simulink model "cartBrick_simulink"  (R2025b)
settings: Solver=ode45  StartTime=0.0  StopTime=10  RelTol=1e-3
values from neighbouring files (symbols this model uses):
  N = 20    [cart_brick_ocp.m]
  nu = length(model.u)    [cart_brick_ocp.m]
undefined symbols (not defined in the file or in its folder): X, Y, Z
libraries: sm_lib x14, nesl_utility x7, simulink x1
settings Model: Creator=oj  LastModifiedBy=itsan
settings SolverCC: AlgebraicLoopSolver=TrustRegion
settings DataIOCC: SaveFormat=StructureWithTime
settings OptimizationCC: LifeSpan=inf
settings DebuggingCC: UnconnectedInputMsg=warning  UnconnectedOutputMsg=warning  UnconnectedLineMsg=warning  SFExecutionAtInitializationDiag=none  ArithmeticOperatorsInVariantConditions=warning
settings HardwareCC: ProdBitPerSizeT=32.0  ProdBitPerPtrDiffT=32.0  ProdWordSize=32.0  ProdHWDeviceType=Specified
settings SFSimCC: CustomCodeUndefinedFunction=UseInterfaceOnly
settings RTWCC: GPUComputeCapability=3.5
settings CodeAppCC: StateflowObjectComments=on

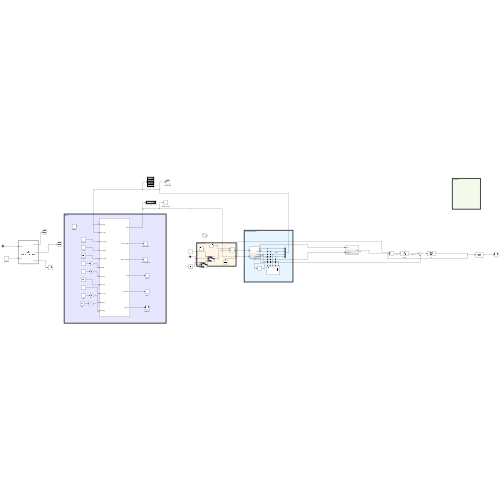
[thumbnail: Simulink's stored preview of the top-level diagram]
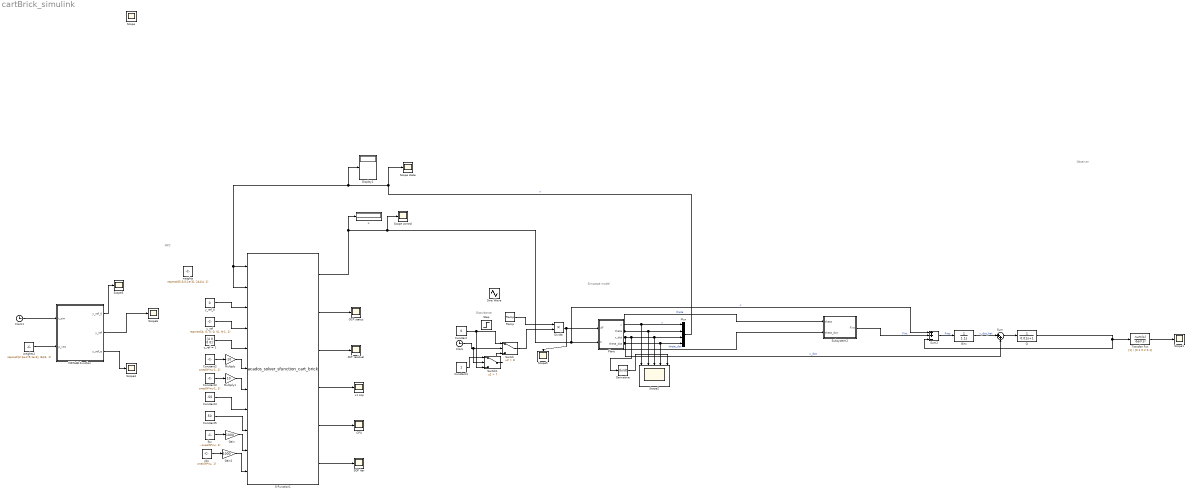
== system cartBrick_simulink ==
  note: Simscape model
  note: Observer
  note: Disturbance
  note: MPC
  CPU : Scope
      settings: Description=status  ActiveDisplayYMinimum=4.7875000000000012E-5  ActiveDisplayYMaximum=0.000858125  DataLoggingVariableName=ScopeData3
  Clock : Clock
      settings: Decimation=7
  Clock1 : Clock
  Constant : Constant  Value=0
  Constant1 : Constant
  Constant2 : Constant  Value=ones(N*nu-1, 1)
  Constant3 : Constant  Value=ones(N*nu-1, 1)
  Constant4 : Constant  Value=-50
  Constant5 : Constant  Value=50
  Derivative : Derivative
  Display1 : Display
  Divide : Product  Inputs=**
  Gain : Gain  Gain=1000
  Gain1 : Gain  Gain=1000
  Ginv : TransferFcn  Denominator=[1.1 0]
  KKT residual : Scope
      settings: Description=status  ActiveDisplayYMinimum=-0.32883901659053916  ActiveDisplayYMaximum=1.592767698176573  DataLoggingVariableName=ScopeData4
  MATLAB Function : MATLAB Function  TreatAsAtomicUnit=on
  Multiply : Gain  Gain=-10
  Multiply1 : Gain  Gain=10
  Mux : Mux
  OCP status : Scope
      settings: Description=status  ActiveDisplayYMinimum=-2.0851401210050069  ActiveDisplayYMaximum=5.2280116787993132
  Plant : Subsystem
  Q : TransferFcn  Denominator=[0.01 1]
  Ramp : simulink/Sources/Ramp  slope=1  start=1  InitialOutput=0
  S-Function1 : S-Function  FunctionName=acados_solver_sfunction_cart_brick  SFunctionDeploymentMode=off  EnableBusSupport=off
      mask Display:
      | % from the make_sfun file
      | global sfun_input_names sfun_output_names
      | for i = 1:length(sfun_input_names)
      | 	port_label('input', i, sfun_input_names{i})
      | end
      | for i = 1:length(sfun_output_names)
      | 	port_label('output', i, sfun_output_names{i})
      | end
  SQP iter : Scope
      settings: Description=status  ActiveDisplayYMinimum=0.875  ActiveDisplayYMaximum=2.125  DataLoggingVariableName=ScopeData5
  Scope control : Scope
      settings: ActiveDisplayYMinimum=-505.22988338563073  ActiveDisplayYMaximum=1195.552745234269  DataLoggingVariableName=ScopeData6
  Scope state : Scope
      settings: ActiveDisplayYMinimum=-0.21964245596561607  ActiveDisplayYMaximum=0.1960092178367589  DataLoggingVariableName=ScopeData7
  Scope{,1,3..6} (6 alike) : Scope
      Scope1 settings: ActiveDisplayYMinimum=-1  ActiveDisplayYMaximum=1  DataLoggingVariableName=ScopeData8
      Scope3 settings: ActiveDisplayYMinimum=-1.7541433017886874  ActiveDisplayYMaximum=4.946334901336316  DataLoggingVariableName=ScopeData10
      Scope4 settings: ActiveDisplayYMinimum=-1.7541433017886874  ActiveDisplayYMaximum=4.946334901336316  DataLoggingVariableName=ScopeData11
      Scope5 settings: ActiveDisplayYMinimum=-1.183238458570643  ActiveDisplayYMaximum=1.630962386741857  DataLoggingVariableName=ScopeData12
      Scope6 settings: ActiveDisplayYMinimum=-1.7541433017886874  ActiveDisplayYMaximum=4.946334901336316  DataLoggingVariableName=ScopeData13
      Scope settings: ActiveDisplayYMinimum=-13.79726  ActiveDisplayYMaximum=10.28583
  Scope2 : Scope  NumInputPorts=5
      settings: ActiveDisplayYMinimum=-14.024186405885914  ActiveDisplayYMaximum=38.526811919180453  DataLoggingVariableName=ScopeData9
  Sine Wave : Sin  Frequency=6*pi  SampleTime=0
  Step : Step  Before=3  After=0  SampleTime=0
  Subsystem2 : Subsystem
  Sum : Sum  Inputs=|++
  Sum2 : Sum  Inputs=+|+|-
  Switch : Switch  Criteria=u2 > Threshold  Threshold=8  SaturateOnIntegerOverflow=off  InputSameDT=off
  Switch1 : Switch  Criteria=u2 > Threshold  Threshold=7  SaturateOnIntegerOverflow=off  InputSameDT=off
  Transfer Fcn : TransferFcn  Denominator=[0.1 0.2 0.1]
  lbu : Constant  Value=- ones(N*nu, 1)
  u : Display
  ubu : Constant  Value=ones(N*nu, 1)
  weights : Constant  Value=repmat([5;3;0;1e-3], 244/4, 1)
  weights1 : Constant  Value=repmat([2;1e-2;5;1e-2], 84/4, 1)
  x1 ocp : Scope
      settings: Description=status  ActiveDisplayYMinimum=-2.6422889921421415  ActiveDisplayYMaximum=2.2266101006407979  DataLoggingVariableName=ScopeData2
  y_ref : Constant  Value=repmat([4; 0; 0; 0; 0], N-1, 1)
  y_ref = 1 : Constant  Value=[4 0 0 0]'
  y_ref_0 : Constant  Value=0
  wires:
  S-Function1/5 -> CPU/1
  S-Function1/6 -> SQP iter/1
  S-Function1/3 -> KKT residual/1
  Mux/1 -> Display1/1, S-Function1/2, S-Function1/1, Scope state/1  "x"
  lbu/1 -> Gain/1
  S-Function1/4 -> x1 ocp/1
  S-Function1/2 -> OCP status/1
  Plant/1(x) -> Mux/1, Scope2/1  "x"
  Plant/3(x_dot) -> Sum/2, Derivative/1, Mux/3, Scope2/3  "x_dot"
  Clock/1 -> Switch1/2, Switch/2
  Constant/1 -> Switch1/3, Switch/1
  Divide/1 -> Plant/1(dF), Scope5/1
  Switch/1 -> Divide/2
  ubu/1 -> Gain1/1
  Constant2/1 -> Multiply/1
  Constant3/1 -> Multiply1/1
  Plant/2(theta) -> Subsystem2/1(theta), Mux/2, Scope2/2  "theta"
  S-Function1/1 -> u/1, Sum2/1, Plant/2(F), Scope control/1  "u"
  Plant/4(theta_dot) -> Subsystem2/2(theta_dot), Mux/4, Scope2/4  "theta_dot"
  Subsystem2/1(Fint) -> Sum2/2  "Fint"
  Q/1 -> Transfer Fcn/1, Sum2/3
  Sum2/1 -> Ginv/1  "Fres"
  Ginv/1 -> Sum/1  "x_dot_hat"
  Sum/1 -> Q/1
  Transfer Fcn/1 -> Scope1/1
  Derivative/1 -> Scope2/5
  Switch1/1 -> Switch/3
  Constant1/1 -> Switch1/1
  Clock1/1 -> MATLAB Function/1(t_sim)
  MATLAB Function/1(y_ref_0) -> Scope3/1
  MATLAB Function/2(y_ref) -> Scope6/1
  MATLAB Function/3(y_ref_e) -> Scope4/1
  weights1/1 -> MATLAB Function/2(p_vec)
  Gain1/1 -> S-Function1/11
  Gain/1 -> S-Function1/10
  Constant5/1 -> S-Function1/9
  Constant4/1 -> S-Function1/8
  Multiply1/1 -> S-Function1/7
  Multiply/1 -> S-Function1/6
  y_ref = 1/1 -> S-Function1/5
  y_ref_0/1 -> S-Function1/3
  y_ref/1 -> S-Function1/4
  Ramp/1 -> Divide/1

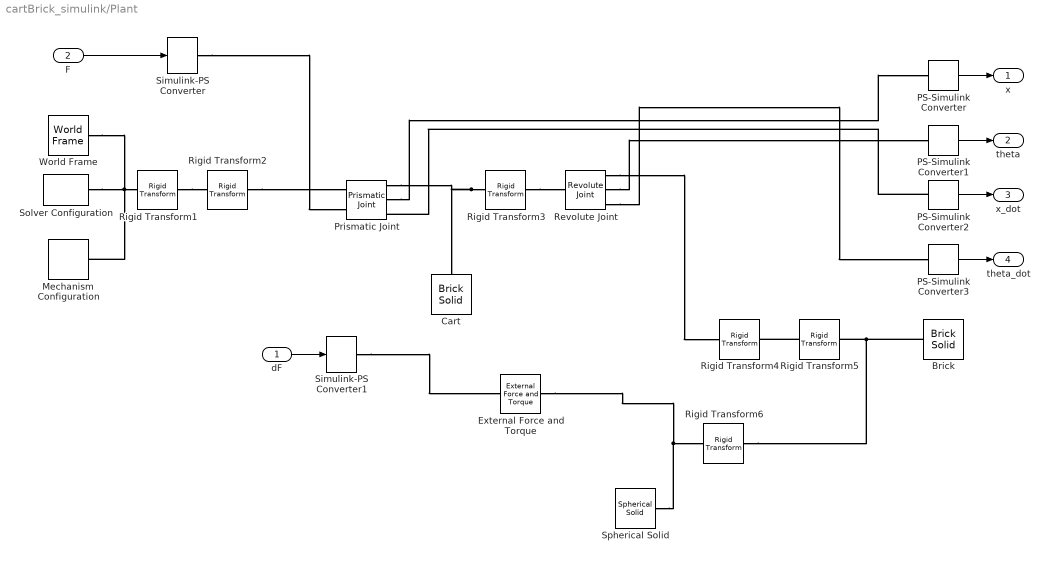
== system cartBrick_simulink/Plant ==
  dF : Inport
  F : Inport  Port=2
  Brick : sm_lib/Body Elements/Brick Solid  BrickDimensions=[0.3 0.8 1]  BrickDimensionsUnits=m  ExportEntireGeometry=off  InertiaType=CalculateFromGeometry  BasedOnType=Mass  Density=1000  DensityUnits=kg/(m^3)  Mass=6  MassUnits=kg  CenterOfMass=[0 0 0]  CenterOfMassUnits=m  MomentsOfInertia=[1 1 1]  MomentsOfInertiaUnits=kg*m^2  ProductsOfInertia=[0 0 0]  ProductsOfInertiaUnits=kg*m^2  GraphicType=FromGeometry  MarkerShape=Sphere  MarkerSize=10  GraphicVisPropType=SimpleVisualProperties  GraphicDiffuseColor=[0.8 0.0 0.2]  GraphicOpacity=0.6  GraphicSpecularColor=[0.5 0.5 0.5 1.0]  GraphicAmbientColor=[0.15 0.15 0.15 1.0]  GraphicEmissiveColor=[0.0 0.0 0.0 1.0]  GraphicShininess=75  DoExposeReferenceFrame=off  SerializedFrames=|
      | <Frames>
      | 
      |   <Frame>
      |     <Id>Frame2</Id>
      |     <Value>
      |       <Name>B</Name>
      |       <Origin>
      |         <Source>GeometricFeature</Source>
      |         <FeatureName>-z surface</FeatureName>
      |       </Origin>
      |       <PrimaryAxis>
      |         <DefinedDirection>+Z</DefinedDirection>
      |         <Source>ReferenceFrame</Source>
      |         <SourceDirection>+Z</SourceDirection>
      |         <FeatureName></FeatureName>
      |       </PrimaryAxis>
      |       <SecondaryAxis>
      |         <DefinedDirection>+X</DefinedDirection>
      |         <Source>ReferenceFrame</Source>
      |         <SourceDirection>+X</SourceDirection>
      |         <FeatureName></FeatureName>
      |       </SecondaryAxis>
      |     </Value>
      |   </Frame>
      | 
      | </Frames>
  Cart : sm_lib/Body Elements/Brick Solid  BrickDimensions=[0.3 0.3 0.3]  BrickDimensionsUnits=m  ExportEntireGeometry=off  InertiaType=PointMass  BasedOnType=Mass  Density=1000  DensityUnits=kg/(m^3)  Mass=10  MassUnits=kg  CenterOfMass=[0 0 0]  CenterOfMassUnits=m  MomentsOfInertia=[1 1 1]  MomentsOfInertiaUnits=kg*m^2  ProductsOfInertia=[0 0 0]  ProductsOfInertiaUnits=kg*m^2  GraphicType=FromGeometry  MarkerShape=Sphere  MarkerSize=10  GraphicVisPropType=SimpleVisualProperties  GraphicDiffuseColor=[0.5 0.5 0.5]  GraphicOpacity=0.5  GraphicSpecularColor=[0.5 0.5 0.5 1.0]  GraphicAmbientColor=[0.15 0.15 0.15 1.0]  GraphicEmissiveColor=[0.0 0.0 0.0 1.0]  GraphicShininess=75  DoExposeReferenceFrame=on  SerializedFrames=<Frames/>
  External Force and Torque : sm_lib/Forces and Torques/External Force and Torque  EnableForceX=on  EnableForceY=off  EnableForceZ=off  EnableForce=off  ForceResolutionFrame=World  EnableTorqueX=off  EnableTorqueY=off  EnableTorqueZ=off  EnableTorque=off  TorqueResolutionFrame=AttachedFrame
  Mechanism Configuration : sm_lib/Utilities/Mechanism Configuration  UniformGravity=Constant  GravityVector=[0 0 -9.81]  GravityVectorUnits=m/s^2  LinearizationDelta=0.001  JointModeTransitionNonlinearIterations=2
  PS-Simulink Converter{,1..3} (4 alike) : nesl_utility/PS-Simulink Converter  PhysicalDomain=network_engine_domain  SubClassName=ps_output  LeftPortType=input  RightPortType=output  PseudoPeriodic=off  Frequencies=[]  VectorFormat=1-D array  Unit=1  AffineConversion=off
  Prismatic Joint : sm_lib/Joints/Prismatic Joint  JointMode=Normal  CompositeWrenchDir=BaseOnFollower  CompositeWrenchFrame=BaseFrame  SenseConstraintForce=off  SenseConstraintTorque=off  SenseTotalForce=off  SenseTotalTorque=off  PositionTargetSpecify=off  PositionTargetPriority=High  PositionTargetValue=0  PositionTargetValueUnits=m  VelocityTargetSpecify=off  VelocityTargetPriority=High  VelocityTargetValue=0  VelocityTargetValueUnits=m/s  EquilibriumPosition=0  EquilibriumPositionUnits=m  SpringStiffness=0  SpringStiffnessUnits=N/m  DampingCoefficient=0  DampingCoefficientUnits=N/(m/s)  LowerLimitSpecify=off  LowerLimitBound=-1  LowerLimitBoundUnits=m  LowerLimitStiffness=1e6  LowerLimitStiffnessUnits=N/m  LowerLimitDamping=1e3  LowerLimitDampingUnits=N/(m/s)  LowerLimitTransitionRegionWidth=1e-4  LowerLimitTransitionRegionWidthUnits=m  UpperLimitSpecify=off  UpperLimitBound=1  UpperLimitBoundUnits=m  UpperLimitStiffness=1e6  UpperLimitStiffnessUnits=N/m  UpperLimitDamping=1e3  UpperLimitDampingUnits=N/(m/s)  UpperLimitTransitionRegionWidth=1e-4  UpperLimitTransitionRegionWidthUnits=m  TorqueActuationMode=InputTorque  MotionActuationMode=ComputedMotion  SensePosition=on  SenseVelocity=on  SenseAcceleration=off  SenseTorqueForce=off  SenseLowerLimitTorqueForce=off  SenseUpperLimitTorqueForce=off
  Revolute Joint : sm_lib/Joints/Revolute Joint  JointMode=Normal  CompositeWrenchDir=FollowerOnBase  CompositeWrenchFrame=BaseFrame  SenseConstraintForce=off  SenseConstraintTorque=off  SenseTotalForce=off  SenseTotalTorque=off  PositionTargetSpecify=on  PositionTargetPriority=High  PositionTargetValue=0  PositionTargetValueUnits=deg  VelocityTargetSpecify=off  VelocityTargetPriority=High  VelocityTargetValue=0  VelocityTargetValueUnits=deg/s  EquilibriumPosition=0  EquilibriumPositionUnits=deg  SpringStiffness=0  SpringStiffnessUnits=N*m/deg  DampingCoefficient=0  DampingCoefficientUnits=N*m/(rad/s)  LowerLimitSpecify=on  LowerLimitBound=-90  LowerLimitBoundUnits=deg  LowerLimitStiffness=1e4  LowerLimitStiffnessUnits=N*m/deg  LowerLimitDamping=10  LowerLimitDampingUnits=N*m/(deg/s)  LowerLimitTransitionRegionWidth=0.1  LowerLimitTransitionRegionWidthUnits=deg  UpperLimitSpecify=on  UpperLimitBound=90  UpperLimitBoundUnits=deg  UpperLimitStiffness=1e4  UpperLimitStiffnessUnits=N*m/deg  UpperLimitDamping=10  UpperLimitDampingUnits=N*m/(deg/s)  UpperLimitTransitionRegionWidth=0.1  UpperLimitTransitionRegionWidthUnits=deg  TorqueActuationMode=NoTorque  MotionActuationMode=ComputedMotion  SensePosition=on  SenseVelocity=on  SenseAcceleration=off  SenseTorqueForce=off  SenseLowerLimitTorqueForce=off  SenseUpperLimitTorqueForce=off
  Rigid Transform1 : sm_lib/Frames and Transforms/Rigid Transform  RotationMethod=StandardAxis  FollAlignAxisA=+X  BaseAlignAxisA=+Y  FollAlignAxisB=+Y  BaseAlignAxisB=+Z  RotationStandardAxis=+Y  RotationAngle=90  RotationAngleUnits=deg  RotationArbitraryAxis=[0 0 1]  RotationSequenceAxes=FollowerAxes  RotationSequence=XYX  RotationSequenceAngles=[0 0 0]  RotationSequenceAnglesUnits=deg  RotationMatrix=[1 0 0; 0 1 0; 0 0 1]  Quaternion=[1 0 0 0]  TranslationMethod=None  TranslationCartesianOffset=[0 0 0]  TranslationCartesianOffsetUnits=m  TranslationStandardAxis=+Z  TranslationStandardOffset=0  TranslationStandardOffsetUnits=m  TranslationROffset=0  TranslationROffsetUnits=m  TranslationThetaOffset=0  TranslationThetaOffsetUnits=deg  TranslationZOffset=0  TranslationZOffsetUnits=m
  Rigid Transform2 : sm_lib/Frames and Transforms/Rigid Transform  RotationMethod=StandardAxis  FollAlignAxisA=+X  BaseAlignAxisA=+Y  FollAlignAxisB=+Y  BaseAlignAxisB=+Z  RotationStandardAxis=+Z  RotationAngle=180  RotationAngleUnits=deg  RotationArbitraryAxis=[0 0 1]  RotationSequenceAxes=FollowerAxes  RotationSequence=XYX  RotationSequenceAngles=[0 0 0]  RotationSequenceAnglesUnits=deg  RotationMatrix=[1 0 0; 0 1 0; 0 0 1]  Quaternion=[1 0 0 0]  TranslationMethod=None  TranslationCartesianOffset=[0 0 0]  TranslationCartesianOffsetUnits=m  TranslationStandardAxis=+Z  TranslationStandardOffset=0  TranslationStandardOffsetUnits=m  TranslationROffset=0  TranslationROffsetUnits=m  TranslationThetaOffset=0  TranslationThetaOffsetUnits=deg  TranslationZOffset=0  TranslationZOffsetUnits=m
  Rigid Transform3 : sm_lib/Frames and Transforms/Rigid Transform  RotationMethod=StandardAxis  FollAlignAxisA=+X  BaseAlignAxisA=+Y  FollAlignAxisB=+Y  BaseAlignAxisB=+Z  RotationStandardAxis=+X  RotationAngle=90  RotationAngleUnits=deg  RotationArbitraryAxis=[0 0 1]  RotationSequenceAxes=FollowerAxes  RotationSequence=XYX  RotationSequenceAngles=[0 0 0]  RotationSequenceAnglesUnits=deg  RotationMatrix=[1 0 0; 0 1 0; 0 0 1]  Quaternion=[1 0 0 0]  TranslationMethod=None  TranslationCartesianOffset=[0 0 0]  TranslationCartesianOffsetUnits=m  TranslationStandardAxis=+Z  TranslationStandardOffset=0  TranslationStandardOffsetUnits=m  TranslationROffset=0  TranslationROffsetUnits=m  TranslationThetaOffset=0  TranslationThetaOffsetUnits=deg  TranslationZOffset=0  TranslationZOffsetUnits=m
  Rigid Transform4 : sm_lib/Frames and Transforms/Rigid Transform  RotationMethod=StandardAxis  FollAlignAxisA=+X  BaseAlignAxisA=+Y  FollAlignAxisB=+Y  BaseAlignAxisB=+Z  RotationStandardAxis=-X  RotationAngle=90  RotationAngleUnits=deg  RotationArbitraryAxis=[0 0 1]  RotationSequenceAxes=FollowerAxes  RotationSequence=XYX  RotationSequenceAngles=[0 0 0]  RotationSequenceAnglesUnits=deg  RotationMatrix=[0 0 1; 0 1 0; 1 0 0]  Quaternion=[1 0 0 0]  TranslationMethod=None  TranslationCartesianOffset=[0 0 0]  TranslationCartesianOffsetUnits=m  TranslationStandardAxis=+Z  TranslationStandardOffset=0  TranslationStandardOffsetUnits=m  TranslationROffset=0  TranslationROffsetUnits=m  TranslationThetaOffset=0  TranslationThetaOffsetUnits=deg  TranslationZOffset=0  TranslationZOffsetUnits=m
  Rigid Transform5 : sm_lib/Frames and Transforms/Rigid Transform  RotationMethod=StandardAxis  FollAlignAxisA=+X  BaseAlignAxisA=+Y  FollAlignAxisB=+Y  BaseAlignAxisB=+Z  RotationStandardAxis=+Y  RotationAngle=90  RotationAngleUnits=deg  RotationArbitraryAxis=[0 0 1]  RotationSequenceAxes=FollowerAxes  RotationSequence=XYX  RotationSequenceAngles=[0 0 0]  RotationSequenceAnglesUnits=deg  RotationMatrix=[0 0 1; 0 1 0; 1 0 0]  Quaternion=[1 0 0 0]  TranslationMethod=None  TranslationCartesianOffset=[0 0 0]  TranslationCartesianOffsetUnits=m  TranslationStandardAxis=+Z  TranslationStandardOffset=0  TranslationStandardOffsetUnits=m  TranslationROffset=0  TranslationROffsetUnits=m  TranslationThetaOffset=0  TranslationThetaOffsetUnits=deg  TranslationZOffset=0  TranslationZOffsetUnits=m
  Rigid Transform6 : sm_lib/Frames and Transforms/Rigid Transform  RotationMethod=None  FollAlignAxisA=+X  BaseAlignAxisA=+Y  FollAlignAxisB=+Y  BaseAlignAxisB=+Z  RotationStandardAxis=+Y  RotationAngle=90  RotationAngleUnits=deg  RotationArbitraryAxis=[0 0 1]  RotationSequenceAxes=FollowerAxes  RotationSequence=XYX  RotationSequenceAngles=[0 0 0]  RotationSequenceAnglesUnits=deg  RotationMatrix=[0 0 1; 0 1 0; 1 0 0]  Quaternion=[1 0 0 0]  TranslationMethod=StandardAxis  TranslationCartesianOffset=[0 0 0]  TranslationCartesianOffsetUnits=m  TranslationStandardAxis=+Z  TranslationStandardOffset=1  TranslationStandardOffsetUnits=m  TranslationROffset=0  TranslationROffsetUnits=m  TranslationThetaOffset=0  TranslationThetaOffsetUnits=deg  TranslationZOffset=0  TranslationZOffsetUnits=m
  Simulink-PS Converter : nesl_utility/Simulink-PS Converter  PhysicalDomain=network_engine_domain  SubClassName=ps_input  LeftPortType=input  RightPortType=output  PseudoPeriodic=off  Frequencies=[]  NoiseDistribution=none  NoiseParameters=[]  Unit=1  AffineConversion=off  FilteringAndDerivatives=zero  SimscapeFilterOrder=1  InputFilterTimeConstant=0.001  UdotUserProvided=1
  Simulink-PS Converter1 : nesl_utility/Simulink-PS Converter  PhysicalDomain=network_engine_domain  SubClassName=ps_input  LeftPortType=input  RightPortType=output  PseudoPeriodic=off  Frequencies=[]  NoiseDistribution=none  NoiseParameters=[]  Unit=1  AffineConversion=off  FilteringAndDerivatives=zero  SimscapeFilterOrder=1  InputFilterTimeConstant=0.001  UdotUserProvided=1
  Solver Configuration : nesl_utility/Solver Configuration  PhysicalDomain=network_engine_domain  SubClassName=solver  LeftPortType=input  RightPortType=generic  Tones=[]  Harmonics=[]  SimulateNoise=off  Profile=off  UseLocalSampling=off  EnableSwitchedLinearOptims=on  FrequencyDomain=off  UseCCode=off  RelTol=0.001  AbsTol=1e-06  MinStep=1e-09  ToWorkspace=off  RevertToSquareIcSolve=off  NumHomotopyIterations=100  PhasorMode=off  PhasorModeNumHarmonics=1  ConsistencySolver=NEWTON_FTOL  IndexReductionMethod=DerivativeReplacement  DoDC=off  ResidualTolerance=1e-09  ConsistencyTolSource=GLOBAL  ConsistencyAbsTol=0.001  ConsistencyRelTol=0.001  ConsistencyTolFactor=0.001  UseLocalSolver=off  LocalSolverChoice=NE_BACKWARD_EULER_ADVANCER  ResolveIndetEquations=on  FunctionEvalNumThread=1  LocalSolverSampleTime=0.001  DoFixedCost=off  MaxNonlinIter=3  MaxModeIter=2  ComputeImpulses=off  ImpulseIterations=2  LinearAlgebra=Sparse  LinearAlgebraNumThread=0  EquationFormulation=NE_TIME_EF  DelaysMemoryBudget=1024  AutomaticFiltering=on  FilteringTimeConstant=0.001  PartitionStorageMethod=AS_NEEDED  PartitionMemoryBudget=1024  PartitionMethod=FAST  MultibodyUseLocalSolver=off  MultibodyLocalSolverChoice=ODE1  MultibodyLocalSolverSampleTime=0.001
  Spherical Solid : sm_lib/Body Elements/Spherical Solid  SphereRadius=0.1  SphereRadiusUnits=m  ExportEntireGeometry=off  InertiaType=PointMass  BasedOnType=Density  Density=1000  DensityUnits=kg/m^3  Mass=1  MassUnits=kg  CenterOfMass=[0 0 0]  CenterOfMassUnits=m  MomentsOfInertia=[1 1 1]  MomentsOfInertiaUnits=kg*m^2  ProductsOfInertia=[0 0 0]  ProductsOfInertiaUnits=kg*m^2  GraphicType=FromGeometry  MarkerShape=Sphere  MarkerSize=10  GraphicVisPropType=AdvancedVisualProperties  GraphicDiffuseColor=[0.5 0.5 0.5]  GraphicOpacity=1  GraphicSpecularColor=[0.8275 0.8275 0.8275]  GraphicAmbientColor=[0.15 0.15 0.15 1.0]  GraphicEmissiveColor=[0.0 0.0 0.0 1.0]  GraphicShininess=75  DoExposeReferenceFrame=on  SerializedFrames=<Frames/>
  World Frame : sm_lib/Frames and Transforms/World Frame
  x : Outport  VectorParamsAs1DForOutWhenUnconnected=off
  theta : Outport  Port=2  VectorParamsAs1DForOutWhenUnconnected=off
  x_dot : Outport  Port=3  VectorParamsAs1DForOutWhenUnconnected=off
  theta_dot : Outport  Port=4  VectorParamsAs1DForOutWhenUnconnected=off
  wires:
  PS-Simulink Converter1/1 -> theta/1
  PS-Simulink Converter/1 -> x/1
  F/1 -> Simulink-PS Converter/1
  dF/1 -> Simulink-PS Converter1/1
  PS-Simulink Converter2/1 -> x_dot/1
  PS-Simulink Converter3/1 -> theta_dot/1
  connections:
  Rigid Transform3/LConn1 -- Cart/RConn1 -- Prismatic Joint/RConn1
  World Frame/RConn1 -- Solver Configuration/RConn1 -- Rigid Transform1/LConn1 -- Mechanism Configuration/RConn1
  Revolute Joint/RConn1 -- Rigid Transform4/LConn1
  Revolute Joint/RConn2 -- PS-Simulink Converter1/LConn1
  Prismatic Joint/RConn2 -- PS-Simulink Converter/LConn1
  Simulink-PS Converter/RConn1 -- Prismatic Joint/LConn2
  Simulink-PS Converter1/RConn1 -- External Force and Torque/LConn1
  Rigid Transform1/RConn1 -- Rigid Transform2/LConn1
  Rigid Transform2/RConn1 -- Prismatic Joint/LConn1
  Revolute Joint/RConn3 -- PS-Simulink Converter3/LConn1
  PS-Simulink Converter2/LConn1 -- Prismatic Joint/RConn3
  Rigid Transform3/RConn1 -- Revolute Joint/LConn1
  Rigid Transform5/LConn1 -- Rigid Transform4/RConn1
  Brick/LConn1 -- Rigid Transform6/LConn1 -- Rigid Transform5/RConn1
  External Force and Torque/RConn1 -- Spherical Solid/RConn1 -- Rigid Transform6/RConn1

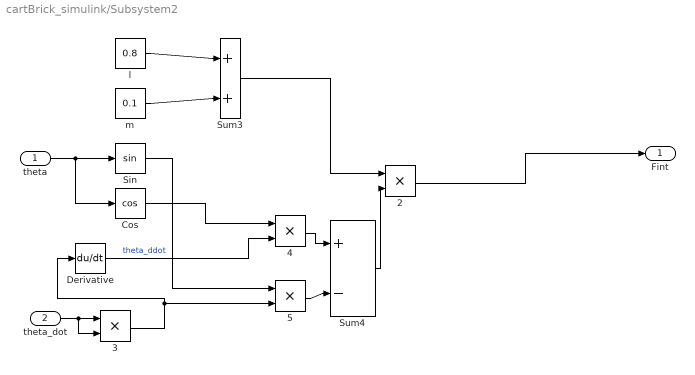
== system cartBrick_simulink/Subsystem2 ==
  theta : Inport
  theta_dot : Inport  Port=2
   {2..5} (4 alike) : Product  Inputs=**
  Cos : Trigonometry  Operator=cos
  Derivative : Derivative
  Sin : Trigonometry
  Sum3 : Sum  Inputs=+|+
  Sum4 : Sum  Inputs=+|-
  l : Constant  Value=0.8
  m : Constant  Value=0.1
  Fint : Outport
  wires:
  " 3"/1 -> Derivative/1, " 5"/2
  Sin/1 -> " 5"/1
  " 5"/1 -> Sum4/2
  " 4"/1 -> Sum4/1
  Sum4/1 -> " 2"/2
  Sum3/1 -> " 2"/1
  l/1 -> Sum3/1
  " 2"/1 -> Fint/1
  theta/1 -> Cos/1, Sin/1
  m/1 -> Sum3/2
  Cos/1 -> " 4"/1
  theta_dot/1 -> " 3"/2, " 3"/1
  Derivative/1 -> " 4"/2  "theta_ddot"

== matlab function cartBrick_simulink/MATLAB Function ==
  data: t_sim input; y_ref_0 output; p_vec input; y_ref output; y_ref_e output
function [y_ref_0, y_ref, y_ref_e] = ramp_reference_inputs(t_sim, p_vec)
% Genera las referencias dinámicas de la rampa para el controlador MPC.
%
% Entradas:
%   t_sim:  Tiempo actual de la simulación.
%   p_vec:  Vector de parámetros online P (pesos Q) del OCP.
%
% Salidas:
%   y_ref_0: Referencia inicial (Control), tamaño [1x1].
%   y_ref:   Referencias intermedias (Estado y Control), tamaño [95x1].
%   y_ref_e: Referencia terminal (Estado), tamaño [4x1].

    % --- Parámetros del OCP ---
    N = 20;            % Numero de pasos del horizonte
    T = 1.0;           % Tiempo total del horizonte
    nx = 4; nu = 1;    % Dimensiones (4 estados, 1 control)
    Ts = T / N;        % Paso de tiempo del OCP (0.05 s)

    % --- Parámetros de la Rampa Deseada ---
    X_FINAL = 4.0;
    T_RAMP = 2.0;      % Tiempo total para alcanzar X_FINAL (2.0 segundos)
    V_RAMP = X_FINAL / T_RAMP;
    
    % --- Vector de Escaldo (asumimos p_vec es constante a lo largo del horizonte) ---
    % En tu setup, p_vec es el vector de pesos p para [x, dx, theta, dtheta]
    
    % Tomamos los primeros 4 elementos de p_vec ya que son los pesos del estado.
    % Usamos la raiz cuadrada para el escalado de la referencia.
    p_weights = p_vec(1:nx, 1);
    sqrt_p = sqrt(p_weights); 
    
    % --- 1. REFERENCIAS INTERMEDIAS (y_ref, tamaño 95x1) ---
    
    % Instantes de tiempo futuros para k=1 a N-1
    time_future = t_sim + (1:(N-1)) * Ts;
    
    % Posición: x(t) = min(t * V_RAMP, X_FINAL)
    x_ref_future = min(time_future * V_RAMP, X_FINAL);
    
    % Velocidad: V_RAMP si aún no termina la rampa, 0 si ya terminó.
    v_ref_future = (time_future <= T_RAMP) * V_RAMP;

    y_ref = zeros((N-1) * (nx + nu), 1);
    
    for k = 1:(N-1)
        
        idx_start = (k-1)*(nx + nu) + 1;
        
        % Estado físico deseado [pos, vel, ang, ang_vel]
        x_ref_fisico = [ 
            x_ref_future(k);
            v_ref_future(k);
            0; 
            0 
        ];
        
        % Escalar el estado físico con sqrt(p)
        ref_x_scaled = sqrt_p .* x_ref_fisico;
        
        % Vector de referencia de 5 elementos: [x_scaled; u]
        step_ref = [ 
            ref_x_scaled; 
            0   % Referencia de control u es 0
        ];
        
        y_ref(idx_start : idx_start + nx + nu - 1, 1) = step_ref;
    end

    % --- 2. REFERENCIA INICIAL (y_ref_0, tamaño 1x1) ---
    % Solo referencia de Control (u), debe ser 0.
    y_ref_0 = 0;

    % --- 3. REFERENCIA TERMINAL (y_ref_e, tamaño 4x1) ---
    
    % El instante de tiempo terminal del horizonte
    t_terminal = t_sim + T; 
    
    % La posición y velocidad física deseada en ese instante terminal
    x_e_fisico = min(t_terminal * V_RAMP, X_FINAL);
    v_e_fisico = (t_terminal <= T_RAMP) * V_RAMP;

    % Estado terminal deseado físico
    x_ref_e_fisico = [x_e_fisico; v_e_fisico; 0; 0];
    
    % y_ref_e DEBE ser el estado terminal ESCALADO
    y_ref_e = sqrt_p .* x_ref_e_fisico;
end
